simulink model "model"  (R2024a)
settings: Solver=VariableStepAuto  StartTime=0.0  StopTime=0.8  RelTol=1e-3
model workspace (MAT data in the model file):
  first_part_line = 200
  second_part_line = 1e-05
libraries: spsFourierLib x8, spsRMSLib x8, spsThreePhasePISectionLineLib x2, spsThreePhaseParallelRLCLoadLib x1, spsThreePhaseVIMeasurementLib x1, spsThreePhaseFaultLib x1, spsThreePhaseSourceLib x1, sps_lib x1
settings Model: Creator=isoko  LastModifiedBy=victor_shapoval

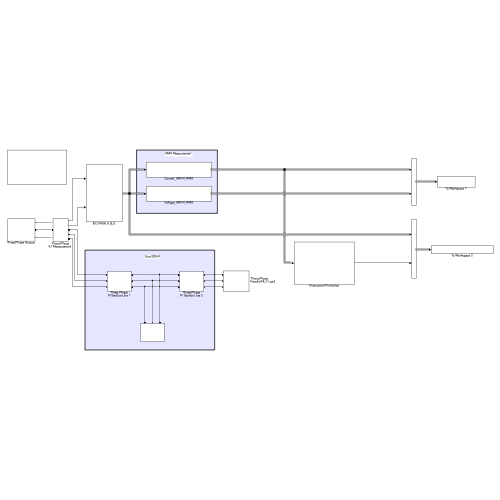
[thumbnail: Simulink's stored preview of the top-level diagram]
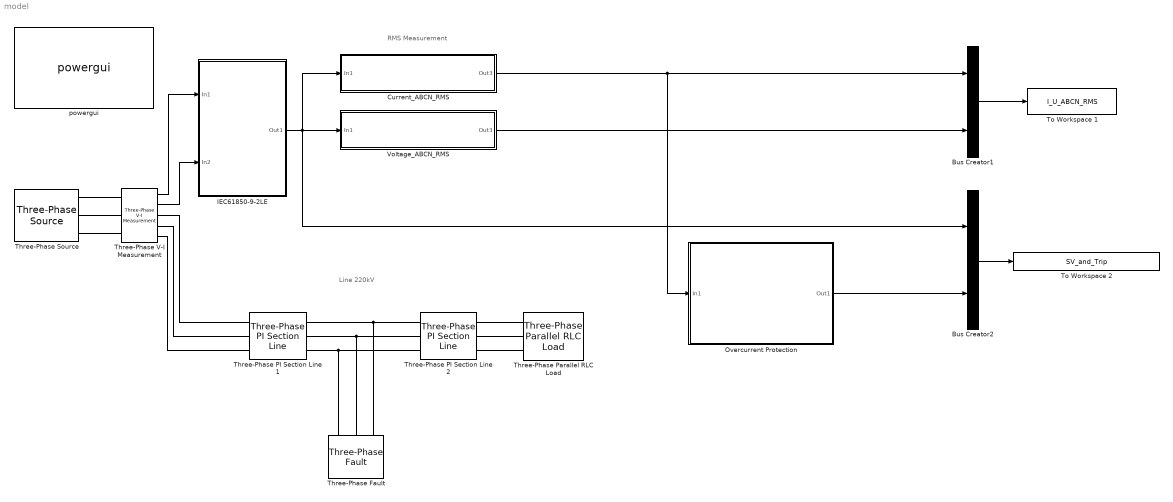
== system model ==
  note: RMS Measurement
  note: Line 220kV
  Bus Creator1 : BusCreator  Inputs=2
  Bus Creator2 : BusCreator  Inputs=2
  Current_ABCN_RMS : Subsystem
  IEC61850-9-2LE : Subsystem
  Overcurrent Protection : Subsystem
  Three-Phase PI Section Line 1 : spsThreePhasePISectionLineLib/Three-Phase PI Section Line  LConnTagsString=a|b|c  RConnTagsString=A|B|C  Length=part1  Frequency=50  Resistances=[0.0703 0.422]  Inductances=[1.336901e-3 3.609e-3]  Capacitances=[8.59755e-9 6.448e-9]
  Three-Phase PI Section Line 2 : spsThreePhasePISectionLineLib/Three-Phase PI Section Line  LConnTagsString=a|b|c  RConnTagsString=A|B|C  Length=part2  Frequency=50  Resistances=[0.0703 0.422]  Inductances=[1.336901e-3 3.609e-3]  Capacitances=[8.59755e-9 6.448e-9]
  "Three-Phase Parallel RLC Load " : spsThreePhaseParallelRLCLoadLib/Three-Phase Parallel RLC Load  LConnTagsString=A|B|C  Configuration=Y (grounded)  NominalVoltage=220e3  Vabc=[1e3 1e3 1e3]  Vabcp=[1e3 1e3 1e3]  NominalFrequency=50  UnbalancedPower=off  ActivePower=100e6  InductivePower=50e6  CapacitivePower=100  Pabc=[10e3 9e3 11e3]  QLabc=[100 90 110]  QCabc=[100 90 110]  Pabcp=[10e3 9e3 11e3]  QLabcp=[100 90 110]  QCabcp=[100 90 110]  Measurements=None  LoadType=constant Z
  "Three-Phase V-I Measurement " : spsThreePhaseVIMeasurementLib/Three-Phase V-I Measurement  VoltageMeasurement=phase-to-ground  SetLabelV=off  LabelV=Vabc  Vpu=off  VpuLL=off  CurrentMeasurement=yes  SetLabelI=off  LabelI=Iabc  Ipu=off  Pbase=100e6  Vbase=230e3  OutputType=Complex  PhasorSimulation=off  PSBequivalent=0
  Three-Phase Fault : spsThreePhaseFaultLib/Three-Phase Fault  InitialStates=0  FaultA=on  FaultB=on  FaultC=on  GroundFault=off  SwitchTimes="[0.45  0.6]"  External=off  SwitchStatus=NaN  FaultResistance=1.2412  GroundResistance=0.001  SnubberResistance=1e6  SnubberCapacitance=inf  Measurements=None
  "Three-Phase Source " : spsThreePhaseSourceLib/Three-Phase Source  InternalConnection=Yg  VoltagePhases=off  Voltage=230e3  PhaseAngle=0  Voltage_phases=[230e3 230e3 230e3]/sqrt(3)  PhaseAngles_phases=[0 -120 +120]  Frequency=50  NonIdealSource=on  SpecifyImpedance=off  Resistance=0.8929  Inductance=16.58e-3  ShortCircuitLevel=100e6  BaseVoltage=230e3  XRratio=7  BusType=swing  Pref=10e3  Qref=0  Prefabc=[10e3, 10e3, 10e3]  Qrefabc=[0, 0, 0]  Qmin=-inf  Qmax=inf
  To Workspace 1 : ToWorkspace  VariableName=I_U_ABCN_RMS  SampleTime=-1
  To Workspace 2 : ToWorkspace  VariableName=SV_and_Trip  SampleTime=-1
  Voltage_ABCN_RMS : Subsystem
  powergui : sps_lib/powergui  Priority=1  SimulationMode=Discrete  SampleTime=50e-6  frequency=60  Iterations=50  frequencyindice=50  Pbase=100e6  ErrMax=1e-4  UnitsV=kV  UnitsW=MW  buscounter=0  FunctionMessages=off  echomessages=on  EnableUseOfTLC=off  CurrentSourceSwitches=off  DisableSnubberDevices=off  DisableRonSwitches=off  DisableVfSwitches=off  DisplayEquations=off  AutomaticDiscreteSolvers=off  SolverType=Tustin/Backward Euler (TBE)  Interpol=off  ExternalGateDelay=off  methode=off  Ts=100  x0status=blocks  SPID=on  SwTol=0  HookPort=off  NonlinearTolerance=1e-4  nMaxIteration=100  ContinueOnMaxIteration=off  RestoreLinks=warning  ResistiveCurrentMeasurement=off  Frange=[0:2:500]  Ylog=off  Xlog=on  ShowGrid=off  save=off  variable=ZData  structure=0  ZoomFFT=off  StartTime=0.0  cycles=1  DisplayStyle=1  fundamental=60  FreqAxis=off  MaxFrequency=1000  frequencyindicesteady=1  RmsSteady=1  display=off
  wires:
  "Three-Phase V-I Measurement "/1 -> IEC61850-9-2LE/1(In1)
  "Three-Phase V-I Measurement "/2 -> IEC61850-9-2LE/2(In2)
  IEC61850-9-2LE/1(Out1) -> Bus Creator2/1, Current_ABCN_RMS/1(In1), Voltage_ABCN_RMS/1(In1)
  Bus Creator2/1 -> To Workspace 2/1
  Current_ABCN_RMS/1(Out3) -> Overcurrent Protection/1(In1), Bus Creator1/1
  Voltage_ABCN_RMS/1(Out3) -> Bus Creator1/2
  Bus Creator1/1 -> To Workspace 1/1
  Overcurrent Protection/1(Out1) -> Bus Creator2/2
  connections:
  "Three-Phase V-I Measurement "/RConn1 -- Three-Phase PI Section Line 1/LConn1
  Three-Phase PI Section Line 1/LConn2 -- "Three-Phase V-I Measurement "/RConn2
  "Three-Phase V-I Measurement "/RConn3 -- Three-Phase PI Section Line 1/LConn3
  "Three-Phase Source "/RConn1 -- "Three-Phase V-I Measurement "/LConn1
  "Three-Phase Source "/RConn2 -- "Three-Phase V-I Measurement "/LConn2
  "Three-Phase Source "/RConn3 -- "Three-Phase V-I Measurement "/LConn3
  Three-Phase PI Section Line 2/RConn1 -- "Three-Phase Parallel RLC Load "/LConn1
  Three-Phase PI Section Line 2/RConn2 -- "Three-Phase Parallel RLC Load "/LConn2
  Three-Phase PI Section Line 2/RConn3 -- "Three-Phase Parallel RLC Load "/LConn3
  Three-Phase PI Section Line 1/RConn1 -- Three-Phase PI Section Line 2/LConn1 -- Three-Phase Fault/LConn1
  Three-Phase PI Section Line 1/RConn2 -- Three-Phase PI Section Line 2/LConn2 -- Three-Phase Fault/LConn2
  Three-Phase PI Section Line 1/RConn3 -- Three-Phase PI Section Line 2/LConn3 -- Three-Phase Fault/LConn3

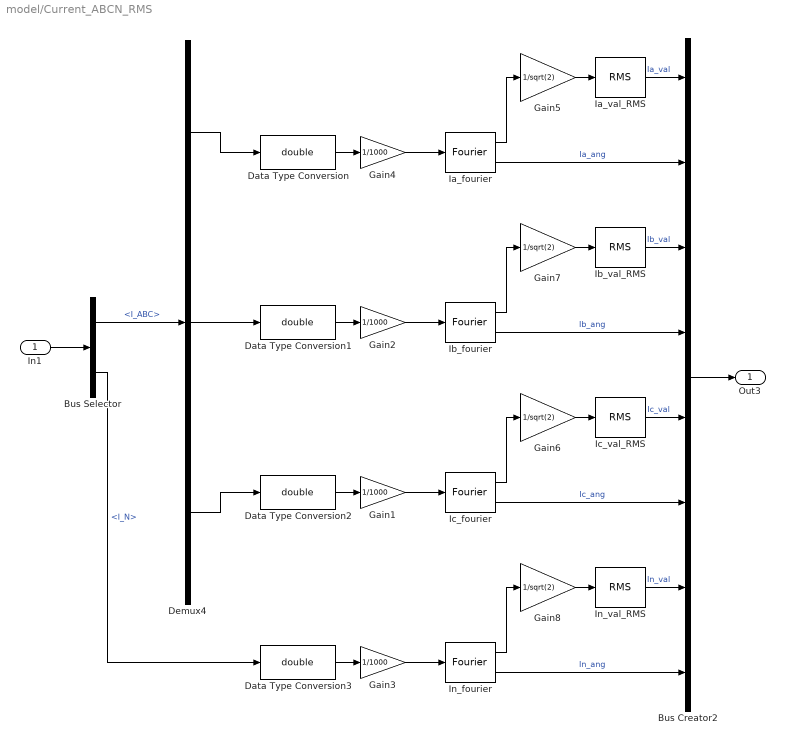
== system model/Current_ABCN_RMS ==
  In1 : Inport
  Bus Creator2 : BusCreator  Inputs=8
  Bus Selector : BusSelector  OutputSignals=I_ABC,I_N
  Data Type Conversion{,1..3} (4 alike) : DataTypeConversion  OutDataTypeStr=double  SaturateOnIntegerOverflow=off  RndMeth=Floor
  Demux4 : Demux  Outputs=3
  Gain{1..4} (4 alike) : Gain  Gain=1/1000  OutDataTypeStr=double
  Gain{5..8} (4 alike) : Gain  Gain=1/sqrt(2)  OutDataTypeStr=double
  Ia_fourier : spsFourierLib/Fourier  Freq=50  n=1  InInit=[0, 0]  Ts=0
  Ia_val_RMS : spsRMSLib/RMS  TrueRMS=on  Freq=50  RMSInit=0  Ts=1/4000
  Ib_fourier : spsFourierLib/Fourier  Freq=50  n=1  InInit=[0, 0]  Ts=0
  Ib_val_RMS : spsRMSLib/RMS  TrueRMS=on  Freq=50  RMSInit=0  Ts=1/4000
  Ic_fourier : spsFourierLib/Fourier  Freq=50  n=1  InInit=[0, 0]  Ts=0
  In_fourier : spsFourierLib/Fourier  Freq=50  n=1  InInit=[0, 0]  Ts=0
  In_val_RMS : spsRMSLib/RMS  TrueRMS=on  Freq=50  RMSInit=0  Ts=1/4000
  Iс_val_RMS : spsRMSLib/RMS  TrueRMS=on  Freq=50  RMSInit=0  Ts=1/4000
  Out3 : Outport
  wires:
  Bus Creator2/1 -> Out3/1
  In_val_RMS/1 -> Bus Creator2/7  "In_val"
  Ib_fourier/2 -> Bus Creator2/4  "Ib_ang"
  Ib_val_RMS/1 -> Bus Creator2/3  "Ib_val"
  Ia_fourier/2 -> Bus Creator2/2  "Ia_ang"
  Ia_val_RMS/1 -> Bus Creator2/1  "Ia_val"
  Data Type Conversion2/1 -> Gain1/1
  Ic_fourier/2 -> Bus Creator2/6  "Iс_ang"
  Gain3/1 -> In_fourier/1
  Gain2/1 -> Ib_fourier/1
  Data Type Conversion3/1 -> Gain3/1
  Data Type Conversion/1 -> Gain4/1
  Iс_val_RMS/1 -> Bus Creator2/5  "Iс_val"
  Demux4/3 -> Data Type Conversion2/1
  In_fourier/2 -> Bus Creator2/8  "In_ang"
  Gain4/1 -> Ia_fourier/1
  Demux4/2 -> Data Type Conversion1/1
  In1/1 -> Bus Selector/1
  Demux4/1 -> Data Type Conversion/1
  Data Type Conversion1/1 -> Gain2/1
  Gain1/1 -> Ic_fourier/1
  Bus Selector/2 -> Data Type Conversion3/1  "<I_N>"
  Bus Selector/1 -> Demux4/1  "<I_ABC>"
  Gain7/1 -> Ib_val_RMS/1
  Ib_fourier/1 -> Gain7/1
  Ia_fourier/1 -> Gain5/1
  Ic_fourier/1 -> Gain6/1
  Gain6/1 -> Iс_val_RMS/1
  In_fourier/1 -> Gain8/1
  Gain8/1 -> In_val_RMS/1
  Gain5/1 -> Ia_val_RMS/1

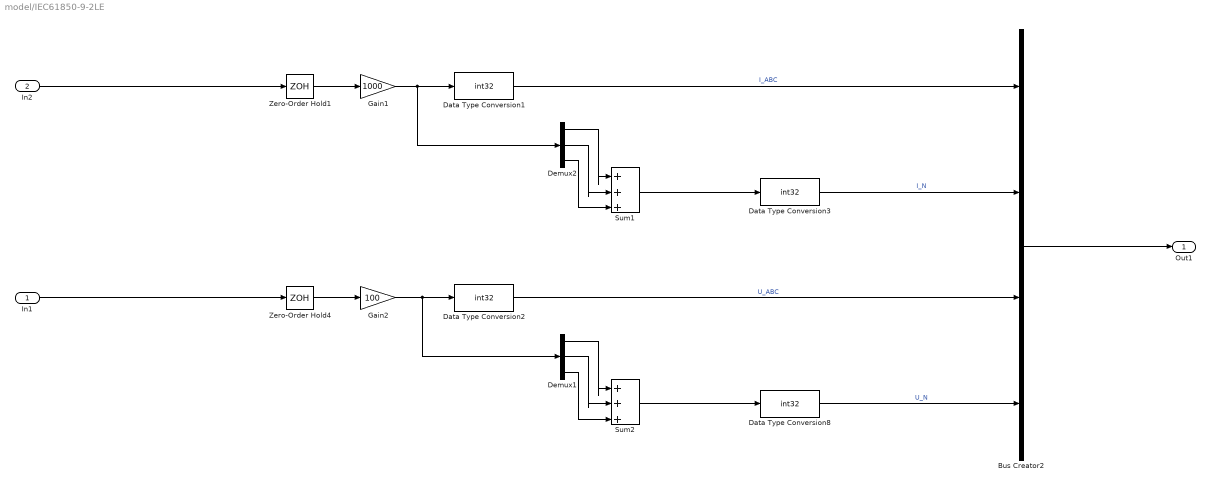
== system model/IEC61850-9-2LE ==
  In1 : Inport
  In2 : Inport  Port=2
  Bus Creator2 : BusCreator  Inputs=4
  Data Type Conversion{1..3,8} (4 alike) : DataTypeConversion  OutDataTypeStr=int32  SaturateOnIntegerOverflow=off  RndMeth=Floor
  Demux1 : Demux  Outputs=3
  Demux2 : Demux  Outputs=3
  Gain1 : Gain  Gain=1000
  Gain2 : Gain  Gain=100
  Sum1 : Sum  Inputs=|+++
  Sum2 : Sum  Inputs=|+++
  Zero-Order Hold1 : ZeroOrderHold  SampleTime=1/4000
  Zero-Order Hold4 : ZeroOrderHold  SampleTime=1/4000
  Out1 : Outport
  wires:
  In2/1 -> Zero-Order Hold1/1
  Zero-Order Hold1/1 -> Gain1/1
  Data Type Conversion8/1 -> Bus Creator2/4  "U_N"
  Demux1/1 -> Sum2/1
  Bus Creator2/1 -> Out1/1
  Sum1/1 -> Data Type Conversion3/1
  Demux1/2 -> Sum2/2
  Demux1/3 -> Sum2/3
  Gain2/1 -> Demux1/1, Data Type Conversion2/1
  In1/1 -> Zero-Order Hold4/1
  Zero-Order Hold4/1 -> Gain2/1
  Gain1/1 -> Demux2/1, Data Type Conversion1/1
  Sum2/1 -> Data Type Conversion8/1
  Data Type Conversion2/1 -> Bus Creator2/3  "U_ABC"
  Data Type Conversion3/1 -> Bus Creator2/2  "I_N"
  Demux2/1 -> Sum1/1
  Demux2/3 -> Sum1/3
  Demux2/2 -> Sum1/2
  Data Type Conversion1/1 -> Bus Creator2/1  "I_ABC"

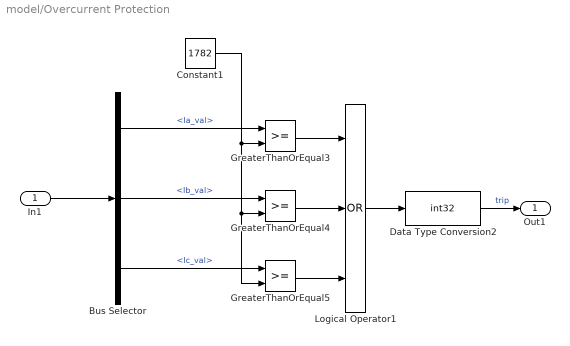
== system model/Overcurrent Protection ==
  In1 : Inport
  Bus Selector : BusSelector  OutputSignals=Ia_val,Ib_val,Iс_val
  Constant1 : Constant  Value=1782
  Data Type Conversion2 : DataTypeConversion  OutDataTypeStr=int32  SaturateOnIntegerOverflow=off  RndMeth=Floor
  GreaterThanOrEqual3 : RelationalOperator  OutDataTypeStr=boolean  RndMeth=Simplest  InputSameDT=off
  GreaterThanOrEqual4 : RelationalOperator  OutDataTypeStr=boolean  RndMeth=Simplest  InputSameDT=off
  GreaterThanOrEqual5 : RelationalOperator  OutDataTypeStr=boolean  RndMeth=Simplest  InputSameDT=off
  Logical Operator1 : Logic  Operator=OR  Inputs=3  AllPortsSameDT=off  OutDataTypeStr=boolean
  Out1 : Outport
  wires:
  In1/1 -> Bus Selector/1
  Logical Operator1/1 -> Data Type Conversion2/1
  GreaterThanOrEqual5/1 -> Logical Operator1/3
  Bus Selector/2 -> GreaterThanOrEqual4/1  "<Ib_val>"
  Data Type Conversion2/1 -> Out1/1  "trip"
  GreaterThanOrEqual3/1 -> Logical Operator1/1
  Constant1/1 -> GreaterThanOrEqual5/2, GreaterThanOrEqual4/2, GreaterThanOrEqual3/2
  Bus Selector/1 -> GreaterThanOrEqual3/1  "<Ia_val>"
  GreaterThanOrEqual4/1 -> Logical Operator1/2
  Bus Selector/3 -> GreaterThanOrEqual5/1  "<Iс_val>"

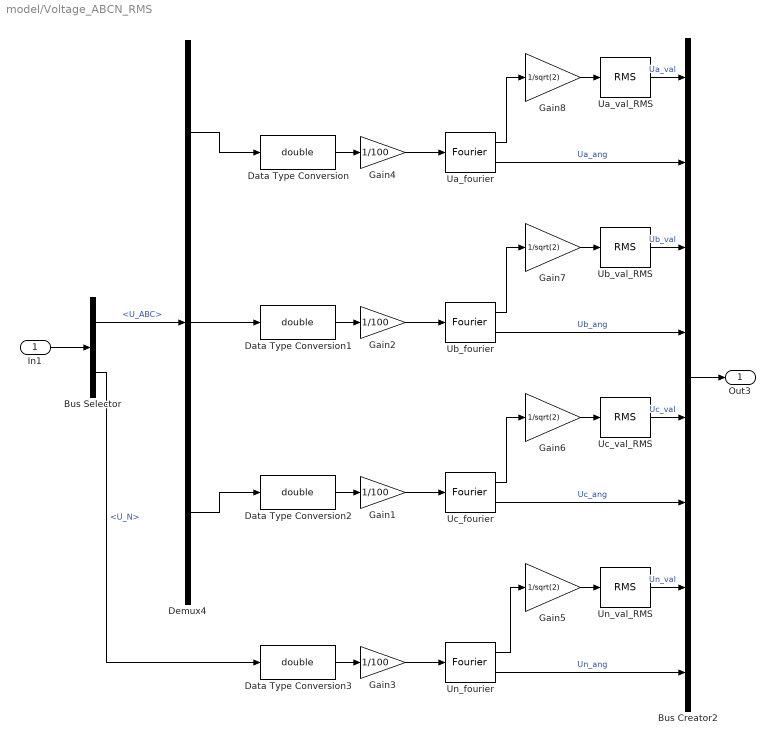
== system model/Voltage_ABCN_RMS ==
  In1 : Inport
  Bus Creator2 : BusCreator  Inputs=8
  Bus Selector : BusSelector  OutputSignals=U_ABC,U_N
  Data Type Conversion{,1..3} (4 alike) : DataTypeConversion  OutDataTypeStr=double  SaturateOnIntegerOverflow=off  RndMeth=Floor
  Demux4 : Demux  Outputs=3
  Gain{1..4} (4 alike) : Gain  Gain=1/100  OutDataTypeStr=double
  Gain{5..8} (4 alike) : Gain  Gain=1/sqrt(2)  OutDataTypeStr=double
  Ua_fourier : spsFourierLib/Fourier  Freq=50  n=1  InInit=[0, 0]  Ts=0
  Ua_val_RMS : spsRMSLib/RMS  TrueRMS=on  Freq=50  RMSInit=0  Ts=1/4000
  Ub_fourier : spsFourierLib/Fourier  Freq=50  n=1  InInit=[0, 0]  Ts=0
  Ub_val_RMS : spsRMSLib/RMS  TrueRMS=on  Freq=50  RMSInit=0  Ts=1/4000
  Uc_fourier : spsFourierLib/Fourier  Freq=50  n=1  InInit=[0, 0]  Ts=0
  Un_fourier : spsFourierLib/Fourier  Freq=50  n=1  InInit=[0, 0]  Ts=0
  Un_val_RMS : spsRMSLib/RMS  TrueRMS=on  Freq=50  RMSInit=0  Ts=1/4000
  Uс_val_RMS : spsRMSLib/RMS  TrueRMS=on  Freq=50  RMSInit=0  Ts=1/4000
  Out3 : Outport
  wires:
  Bus Creator2/1 -> Out3/1
  Un_val_RMS/1 -> Bus Creator2/7  "Un_val"
  Ub_fourier/2 -> Bus Creator2/4  "Ub_ang"
  Ub_val_RMS/1 -> Bus Creator2/3  "Ub_val"
  Ua_fourier/2 -> Bus Creator2/2  "Ua_ang"
  Ua_val_RMS/1 -> Bus Creator2/1  "Ua_val"
  Data Type Conversion2/1 -> Gain1/1
  Ub_fourier/1 -> Gain7/1
  Uc_fourier/2 -> Bus Creator2/6  "Uс_ang"
  Ua_fourier/1 -> Gain8/1
  Gain3/1 -> Un_fourier/1
  Gain2/1 -> Ub_fourier/1
  Data Type Conversion3/1 -> Gain3/1
  Un_fourier/1 -> Gain5/1
  Data Type Conversion/1 -> Gain4/1
  Uс_val_RMS/1 -> Bus Creator2/5  "Uс_val"
  Demux4/3 -> Data Type Conversion2/1
  Un_fourier/2 -> Bus Creator2/8  "Un_ang"
  Gain4/1 -> Ua_fourier/1
  Demux4/2 -> Data Type Conversion1/1
  In1/1 -> Bus Selector/1
  Demux4/1 -> Data Type Conversion/1
  Data Type Conversion1/1 -> Gain2/1
  Gain1/1 -> Uc_fourier/1
  Bus Selector/2 -> Data Type Conversion3/1  "<U_N>"
  Uc_fourier/1 -> Gain6/1
  Bus Selector/1 -> Demux4/1  "<U_ABC>"
  Gain5/1 -> Un_val_RMS/1
  Gain6/1 -> Uс_val_RMS/1
  Gain7/1 -> Ub_val_RMS/1
  Gain8/1 -> Ua_val_RMS/1
